simulink model "Circuit"  (R2017a)
settings: Solver=FixedStepDiscrete  StartTime=0.0  StopTime=0.125 - 5e-5  RelTol=1e-3
libraries: powerlib x11, mylib x2
settings Model: Creator=lefteris  LastModifiedBy=lefteris
settings DataIOCC: SaveTime=off
settings DebuggingCC: UnconnectedInputMsg=none  UnconnectedOutputMsg=none  UnconnectedLineMsg=none

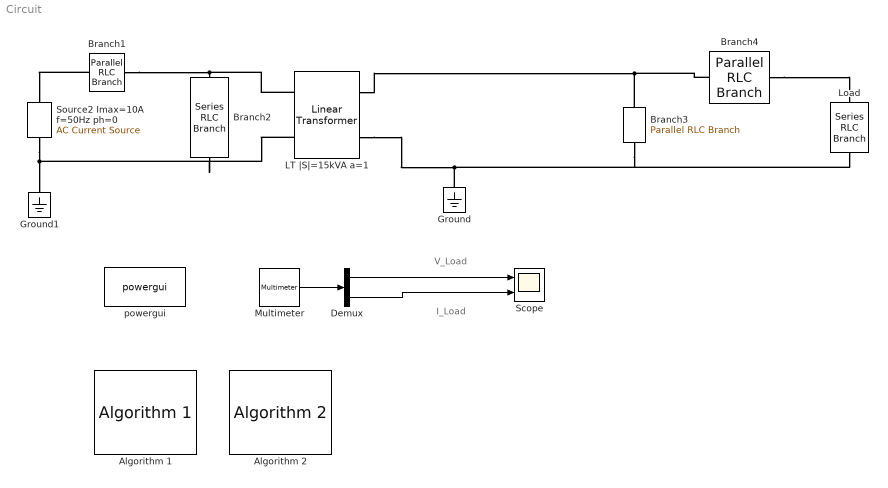
== system Circuit ==
  note: V_Load
  note: I_Load
  Algorithm 1 : mylib/Algorithm 1  SystemSampleTime=-1
      settings: SourceProductName=My Library
  Algorithm 2 : mylib/Algorithm 2  SystemSampleTime=-1
      settings: SourceProductName=My Library
  Branch1 : powerlib/Elements/Parallel RLC Branch  LConnTagsString=a  RConnTagsString=__new0  BranchType=R  Resistance=1000  Inductance=1e-3  SetiL0=off  InitialCurrent=0  Capacitance=1e-6  Setx0=off  InitialVoltage=0  Measurements=None
  Branch2 : powerlib/Elements/Series RLC Branch  LConnTagsString=__new0  RConnTagsString=__new0  BranchType=RC  Resistance=1000  Inductance=1e-3  SetiL0=off  InitialCurrent=0  Capacitance=1e-6  Setx0=off  InitialVoltage=0  Measurements=None
  Branch3 : powerlib/Elements/Parallel RLC Branch  LConnTagsString=a  RConnTagsString=__new0  BranchType=R  Resistance=1000  Inductance=1e-3  SetiL0=off  InitialCurrent=0  Capacitance=1e-6  Setx0=off  InitialVoltage=0  Measurements=None
  Branch4 : powerlib/Elements/Parallel RLC Branch  LConnTagsString=a  RConnTagsString=__new0  BranchType=RL  Resistance=1000  Inductance=1e-3  SetiL0=off  InitialCurrent=0  Capacitance=1e-3  Setx0=off  InitialVoltage=0  Measurements=None
  Demux : Demux  Outputs=2
  Ground : powerlib/Elements/Ground  LConnTagsString=a
  Ground1 : powerlib/Elements/Ground  LConnTagsString=a
  LT |S|=15kVA a=1 : powerlib/Elements/Linear Transformer  UNITS=SI  NominalPower=[15e3 50]  winding1=[220 30 0.1541]  winding2=[220 10 0.10641]  ThreeWindings=off  winding3=[3.15e+05 315.06 0.10641]  RmLm=[1e6 0.5965]  Measurements=None  DataType=on
  Load : powerlib/Elements/Series RLC Branch  LConnTagsString=__new0  RConnTagsString=__new0  BranchType=R  Resistance=2.42  Inductance=0.42  SetiL0=off  InitialCurrent=0  Capacitance=3  Setx0=off  InitialVoltage=0  Measurements=Branch voltage and current
  Multimeter : powerlib/Measurements/Multimeter  PhasorSimulation=off  OutputType=Complex  sel=[1 2]  L=2  Gain=[1 1]  yselected={'Ub: Load','Ib: Load'};  PSBOutputType=1  PSBequivalent=0  AxesSetting=[0,0.1,-100,100]  Display=0  SavedBlockNames=-11
  Scope : Scope  NumInputPorts=2
  Source2 Imax=10A f=50Hz ph=0 : powerlib/Electrical Sources/AC Current Source  Amplitude=10  Phase=0  Frequency=50  SampleTime=0  Measurements=None
      settings: SourceProductName=Simscape Power Systems  SourceProductBaseCode=PS
  powergui : powerlib/powergui  Priority=1  SimulationMode=Discrete  SampleTime=50e-6  frequency=60  Iterations=50  frequencyindice=50  Pbase=100e6  ErrMax=1e-4  UnitsV=kV  UnitsW=MW  buscounter=0  FunctionMessages=off  echomessages=off  EnableUseOfTLC=off  CurrentSourceSwitches=off  DisableSnubberDevices=off  DisableRonSwitches=off  DisableVfSwitches=off  DisplayEquations=off  SolverType=Tustin  Interpol=off  ExternalGateDelay=off  methode=off  Ts=100  x0status=zero  SPID=on  SwTol=0  HookPort=off  RestoreLinks=warning  ResistiveCurrentMeasurement=off  Frange=[0:2:500]  Ylog=off  Xlog=on  ShowGrid=off  save=off  variable=ZData  structure=logsout  ZoomFFT=off  StartTime=0.0  cycles=1  DisplayStyle=1  fundamental=60  FreqAxis=off  MaxFrequency=1000  frequencyindicesteady=1  RmsSteady=1  display=off
  wires:
  Multimeter/1 -> Demux/1
  Demux/1 -> Scope/1
  Demux/2 -> Scope/2
  connections:
  Branch3/RConn1 -- Load/RConn1 -- LT |S|=15kVA a=1/RConn2 -- Ground/LConn1
  Branch1/LConn1 -- LT |S|=15kVA a=1/LConn1 -- Branch2/LConn1
  LT |S|=15kVA a=1/LConn2 -- Branch2/RConn1 -- Source2 Imax=10A f=50Hz ph=0/LConn1 -- Ground1/LConn1
  LT |S|=15kVA a=1/RConn1 -- Branch3/LConn1 -- Branch4/RConn1
  Branch4/LConn1 -- Load/LConn1
  Branch1/RConn1 -- Source2 Imax=10A f=50Hz ph=0/RConn1
